simulink model "avg_model_gov"  (R2018a)
settings: Solver=ode4  StartTime=0.0  StopTime=Ttotal  FixedStep=Ts  RelTol=1e-3
values from neighbouring files (symbols this model uses):
  Dmin = Pb / (rss * (1-rtr))    (= 1.90222222222)    [avg_model_script.m]
  Dtg1 = Dmin/2    (= 0.951111111111)    [avg_model_script.m]
  Dtg2 = Dtg1    (= 0.951111111111)    [avg_model_script.m]
  M = 10.2    [avg_model_script.m]
  Pb = 0.0428    [avg_model_script.m]
  rtr = 0.1    [avg_model_script.m]
  Tgt1 = 0.1    [avg_model_script.m]
  Tgt2 = Tgt1    (= 0.1)    [avg_model_script.m]
  Tstep = 0.5    [avg_model_script.m]
  Ttg1 = 0.1    [avg_model_script.m]
  Ttg2 = Ttg1    (= 0.1)    [avg_model_script.m]
  x0 = 0    [avg_model_script.m]
settings Model: Creator=ericfa  LastModifiedBy=ericfa

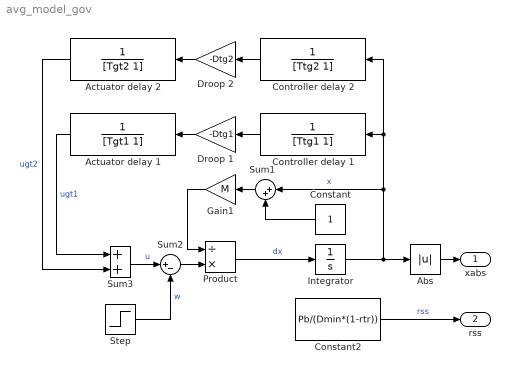
== system avg_model_gov ==
  Abs : Abs
  Actuator delay 1 : TransferFcn  Denominator=[Tgt1 1]
  Actuator delay 2 : TransferFcn  Denominator=[Tgt2 1]
  Constant : Constant
  Constant2 : Constant  Value=Pb/(Dmin*(1-rtr))
  Controller delay 1 : TransferFcn  Denominator=[Ttg1 1]
  Controller delay 2 : TransferFcn  Denominator=[Ttg2 1]
  Droop 1 : Gain  Gain=-Dtg1
  Droop 2 : Gain  Gain=-Dtg2
  Gain1 : Gain  Gain=M
  Integrator : Integrator  InitialCondition=x0
  Product : Product  Inputs=/*
  Step : Step  Time=Tstep  After=Pb  SampleTime=0
  Sum1 : Sum  Inputs=|++
  Sum2 : Sum  Inputs=|+-
  Sum3 : Sum
  xabs : Outport
  rss : Outport  Port=2
  wires:
  Product/1 -> Integrator/1  "dx"
  Integrator/1 -> Abs/1, Controller delay 2/1, Controller delay 1/1, Sum1/1  "x"
  Sum1/1 -> Gain1/1
  Constant/1 -> Sum1/2
  Gain1/1 -> Product/1
  Sum2/1 -> Product/2
  Step/1 -> Sum2/2  "w"
  Constant2/1 -> rss/1  "rss"
  Droop 1/1 -> Actuator delay 1/1
  Controller delay 1/1 -> Droop 1/1
  Abs/1 -> xabs/1
  Sum3/1 -> Sum2/1  "u"
  Actuator delay 1/1 -> Sum3/1  "ugt1"
  Controller delay 2/1 -> Droop 2/1
  Droop 2/1 -> Actuator delay 2/1
  Actuator delay 2/1 -> Sum3/2  "ugt2"
